simulink model "ofdm"  (R2019b)
settings: Solver=VariableStepAuto  StartTime=0.0  StopTime=10000  RelTol=1e-3
undefined symbols (not defined in the file): doppler, EbNo
libraries: commchan3 x3, commdigbbndpm3 x2, commofdm x2, commrandsrc3 x1, commsink2 x1
settings Model: Creator=jose_  LastModifiedBy=jose_

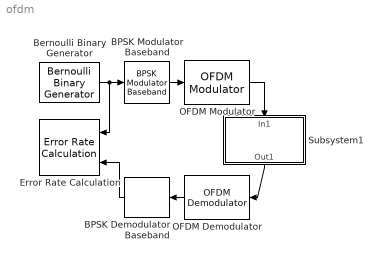
== system ofdm ==
  BPSK Demodulator Baseband : commdigbbndpm3/BPSK Demodulator Baseband  DecType=Hard decision  VarSource=Dialog  Variance=1  Ph=0  outDtype=Inherit via internal rule  derotateFactorWordLen=16  derotateFactorDataTypeStr=Inherit: Same word length as input  derotateFactorLastDataTypeStr=Inherit: Same word length as input
      settings: SourceProductName=Communications Toolbox
  BPSK Modulator Baseband : commdigbbndpm3/BPSK Modulator Baseband  Ph=0  outDtype=double  outWordLen=16  outUDDataType=sfix(16)  outFracLenMode=Best precision  outFracLen=15  outDataTypeStr=double  outLastDataTypeStr=double
      settings: SourceProductName=Communications Toolbox
  Bernoulli Binary Generator : commrandsrc3/Bernoulli Binary Generator  ProbabilityOfZero=0.5  SeedSource=Auto  Seed=0  SampleTime=0.01  SamplesPerFrame=64-11  OutputDataType=double  SimulateUsing=Interpreted execution
      settings: SourceProductName=Communications Toolbox
  Error Rate Calculation : commsink2/Error Rate Calculation  N=0  st_delay=0  cp_mode=Entire frame  subframe=[]  PMode=Workspace  WsName=ErrorVec  RsMode2=off  stop=off  numErr=100  maxBits=1e6
      settings: SourceProductName=Communications Toolbox
  OFDM Demodulator : commofdm/OFDM Demodulator  FFTLength=64  NumGuardBandCarriers=[6; 5]  RemoveDCCarrier=off  PilotOutputPort=off  PilotCarrierIndices=[12; 26; 40; 54]  CyclicPrefixLength=16  NumSymbols=1  NumReceiveAntennas=1  SimulateUsing=Interpreted execution
      settings: SourceProductName=Communications Toolbox  SourceProductBaseCode=CM
  OFDM Modulator : commofdm/OFDM Modulator  FFTLength=64  NumGuardBandCarriers=[6; 5]  InsertDCNull=off  PilotInputPort=off  PilotCarrierIndices=[12; 26; 40; 54]  CyclicPrefixLength=16  Windowing=off  WindowLength=1  NumSymbols=1  NumTransmitAntennas=1  SimulateUsing=Interpreted execution
      settings: SourceProductName=Communications Toolbox  SourceProductBaseCode=CM
  Subsystem1 : Subsystem  mask{Channel_Type=AWGN, AWGN_EbNo=EbNo, AWGN_K=64+16, AWGN_SymbolPeriod=0.01, Ray_delays=0.00001, Ray_Doppler=0.001}
      mask prompts: Channel_Type "Channel Type"; AWGN_EbNo "EbNo (dB)"; AWGN_K "Bits per Symbol"; AWGN_SymbolPeriod "Symbol Period"; Ray_delays "Discrete Path Delays (s)"; Ray_Doppler "Max Doppler Shift (Hz)"
      mask TypeOptions Channel_Type: AWGN | AWGN + Rayleigh
      mask DialogControl AWGN Prompt: AWGN
      mask DialogControl Container7 Prompt: Rayleigh
      mask Display: image('C:\Users\jose_\Pictures\channel.png'); % Use "Edit Image" on toolstrip to change.
  wires:
  OFDM Demodulator/1 -> BPSK Demodulator Baseband/1
  BPSK Modulator Baseband/1 -> OFDM Modulator/1
  Bernoulli Binary Generator/1 -> Error Rate Calculation/1, BPSK Modulator Baseband/1
  BPSK Demodulator Baseband/1 -> Error Rate Calculation/2
  OFDM Modulator/1 -> Subsystem1/1(In1)
  Subsystem1/1(Out1) -> OFDM Demodulator/1

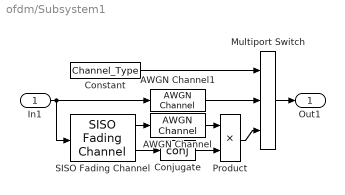
== system ofdm/Subsystem1 ==
  In1 : Inport
  AWGN Channel : commchan3/AWGN Channel  InputProcessing=Columns as channels (frame based)  seed=67  noiseMode="Signal to noise ratio  (Eb/No)"  EbNodB=AWGN_EbNo  EsNodB=10  SNRdB=10  bitsPerSym=AWGN_K  Ps=1  Tsym=AWGN_SymbolPeriod  variance=1
      settings: SourceProductName=Communications Toolbox
  AWGN Channel1 : commchan3/AWGN Channel  InputProcessing=Columns as channels (frame based)  seed=67  noiseMode="Signal to noise ratio  (Eb/No)"  EbNodB=AWGN_EbNo  EsNodB=10  SNRdB=10  bitsPerSym=AWGN_K  Ps=1  Tsym=AWGN_SymbolPeriod  variance=1
      settings: SourceProductName=Communications Toolbox
  Conjugate : Math  Operator=conj  RndMeth=Zero  SaturateOnIntegerOverflow=on
  Constant : Constant  Value=Channel_Type
  Multiport Switch : MultiPortSwitch  Inputs=2
  Product : Product
  SISO Fading Channel : commchan3/SISO Fading Channel  InheritSampleRate=on  SampleRate=1  PathDelays=Ray_delays  AveragePathGains=0  NormalizePathGains=on  FadingDistribution=Rayleigh  KFactor=3  DirectPathDopplerShift=0  DirectPathInitialPhase=0  MaximumDopplerShift=Ray_Doppler  DopplerSpectrum=doppler('Jakes')  RandomStream=mt19937ar with seed  Seed=73  PathGainsOutputPort=on  ChannelFilterDelayOutputPort=off  SimulateUsing=Interpreted execution  Visualization=Off  PathsForDopplerDisplay=1  SamplesToDisplay=25%
      settings: SourceProductName=Communications Toolbox
  Out1 : Outport
  wires:
  Conjugate/1 -> Product/2
  SISO Fading Channel/2 -> Conjugate/1
  In1/1 -> SISO Fading Channel/1, AWGN Channel1/1
  AWGN Channel/1 -> Product/1
  SISO Fading Channel/1 -> AWGN Channel/1
  Multiport Switch/1 -> Out1/1
  Product/1 -> Multiport Switch/3
  AWGN Channel1/1 -> Multiport Switch/2
  Constant/1 -> Multiport Switch/1
